simulink model "Circuit_Overall"  (R2022a)
settings: Solver=VariableStepAuto  StartTime=0.0  StopTime=10.0  RelTol=1e-3
model workspace (MAT data in the model file):
  A_CT = [0  1  0  0; -0.3  -2  0.15  0; 0  0  0  1; 0.15  0  -0.15  0]
  A_ROM = [0.943044110382  0.118843544317  -0.000909529747315  -0.000138540821229; -0.118857686914  -0.0157812554457  -0.0137776836483  -0.00909334104542; -0.0025342762873  0.0670073590662  0.9998525429  -0.00298189729264; -0.000117282969016  0.00874584867536  -0.0147374173206  0.677164807823]
  A_est = [0.943044110382  0.118843544317  -0.000909529747315  -0.000138540821229; -0.118857686914  -0.0157812554457  -0.0137776836483  -0.00909334104542; -0.0025342762873  0.0670073590662  0.9998525429  -0.00298189729264; -0.000117282969016  0.00874584867536  -0.0147374173206  0.677164807823]
  B_CT = [0; 0.2; 0; 0]
  B_ROM = [-0.95489814482; -0.95494703327; -0.000585000179048; 1.23585165252e-07]
  B_est = [-0.95489814482; -0.95494703327; -0.000585000179048; 1.23585165252e-07]
  C = [0 0 1]
  C1 = 10
  C4 = 1000
  C_ROM = [-0.00226305907282 0.00223989493555 0.0376233059802 -0.000112980615776]
  C_est = [-0.00226305907282 0.00223989493555 0.0376233059802 -0.000112980615776]
  F_in = 1
  Iden = [1  0  0  0; 0  1  0  0; 0  0  1  0; 0  0  0  1]
  InputSignal = [0  1; 0.847457627119  1; 1.69491525424  1; 2.54237288136  1; 3.38983050847  1; 4.23728813559  1; 5.08474576271  1; 5.93220338983  1; 6.77966101695  1; 7.62711864407  1; 8.47457627119  1; 9.32203389831  1; 10.1694915254  1; 11.0169491525  1; 11.8644067797  1; 12.7118644068  1; 13.5593220339  1; 14.406779661  1; 15.2542372881  1; 16.1016949153  1; 16.9491525424  1; 17.7966101695  1; 18.6440677966  1; 19.4915254237  1; 20.3389830508  1; 21.186440678  1; 22.0338983051  1; 22.8813559322  1; 23.7288135593  1; 24.5762711864  1; 25.4237288136  1; 26.2711864407  1; 27.1186440678  1; 27.9661016949  1; 28.813559322  1; 29.6610169492  1; 30.5084745763  1; 31.3559322034  1; 32.2033898305  1; 33.0508474576  1; 33.8983050847  1; 34.7457627119  1; 35.593220339  1; 36.4406779661  1; 37.2881355932  1; 38.1355932203  1; 38.9830508475  1; 39.8305084746  1; 40.6779661017  1; 41.5254237288  1; 42.3728813559  1; 43.2203389831  1; 44.0677966102  1; 44.9152542373  1; 45.7627118644  1; 46.6101694915  1; 47.4576271186  1; 48.3050847458  1; 49.1525423729  1; 50  1]
  K_infty = [-1.77627221347; 0.215371488834; 0.631772786096; -0.0204147725383]
  P_k_0 = [0.5  0  0  0; 0  0.5  0  0; 0  0  0.5  0; 0  0  0  0.5]
  Q = 0.1
  R = 0.001
  R1 = 2
  R2 = 2
  R3 = 2
  R4 = 2
  Ts = 1
  Vs = 1
  b = 10
  k1 = 0.75
  k2 = 0.75
  m1 = 5
  m2 = 5
  omega = 0
  x0 = [0; 0; 0; 0]
  x0_2D = [0; 0]
  x0_ROM = [0; 0; 0; 0]
  x0_est = [0; 0; 0; 0]
  x_0_est = [0; 0; 0; 0]
settings Model: Creator=tyevans  LastModifiedBy=tyevans

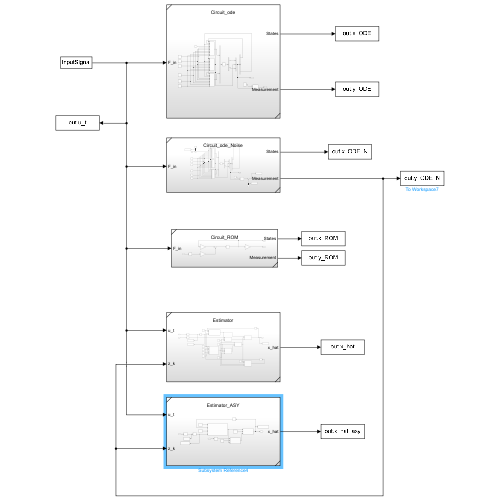
[thumbnail: Simulink's stored preview of the top-level diagram]
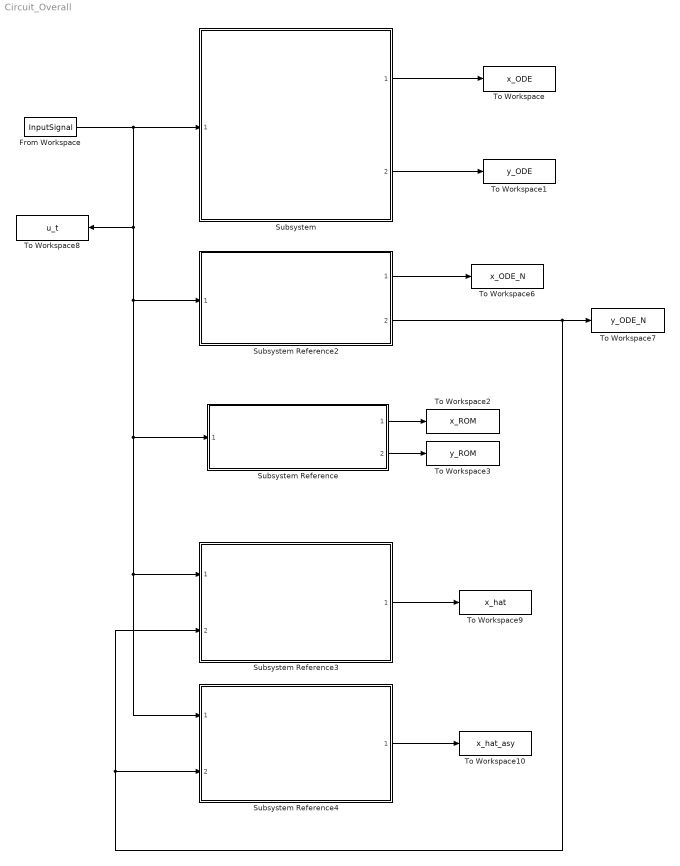
== system Circuit_Overall ==
  From Workspace : FromWorkspace  VariableName=InputSignal  OutputAfterFinalValue=Setting to zero
  Subsystem : Subsystem  ReferencedSubsystem=Circuit_ode
  Subsystem Reference : Subsystem  ReferencedSubsystem=Circuit_ROM
  Subsystem Reference2 : Subsystem  ReferencedSubsystem=Circuit_ode_Noise
  Subsystem Reference3 : Subsystem  ReferencedSubsystem=Estimator
  Subsystem Reference4 : Subsystem  ReferencedSubsystem=Estimator_ASY
  To Workspace : ToWorkspace  VariableName=x_ODE  SaveFormat=Structure With Time  SampleTime=-1
  To Workspace1 : ToWorkspace  VariableName=y_ODE  SaveFormat=Structure With Time  SampleTime=-1
  To Workspace10 : ToWorkspace  VariableName=x_hat_asy  SaveFormat=Structure With Time  SampleTime=-1
  To Workspace2 : ToWorkspace  VariableName=x_ROM  SaveFormat=Structure With Time  SampleTime=-1
  To Workspace3 : ToWorkspace  VariableName=y_ROM  SaveFormat=Structure With Time  SampleTime=-1
  To Workspace6 : ToWorkspace  VariableName=x_ODE_N  SaveFormat=Structure With Time  SampleTime=-1
  To Workspace7 : ToWorkspace  VariableName=y_ODE_N  SaveFormat=Structure With Time  SampleTime=-1
  To Workspace8 : ToWorkspace  VariableName=u_t  SaveFormat=Structure With Time  SampleTime=-1
  To Workspace9 : ToWorkspace  VariableName=x_hat  SaveFormat=Structure With Time  SampleTime=-1
  wires:
  Subsystem/1 -> To Workspace/1
  Subsystem/2 -> To Workspace1/1
  Subsystem Reference2/1 -> To Workspace6/1
  Subsystem Reference3/1 -> To Workspace9/1
  From Workspace/1 -> To Workspace8/1, Subsystem Reference/1, Subsystem Reference4/1, Subsystem Reference3/1, Subsystem Reference2/1, Subsystem/1
  Subsystem Reference2/2 -> Subsystem Reference4/2, Subsystem Reference3/2, To Workspace7/1
  Subsystem Reference4/1 -> To Workspace10/1
  Subsystem Reference/1 -> To Workspace2/1
  Subsystem Reference/2 -> To Workspace3/1
